simulink subsystem "aero_body_normal"  (R2026a)
settings: Solver=VariableStepAuto
undefined symbols (not defined in the file or in its folder): body_area_aft, body_area_bow, body_area_planform, body_length, body_pos_x_cp, body_volume, nosecone_area_aft, nosecone_area_bow, nosecone_area_planform, nosecone_length, nosecone_pos_x_cp, nosecone_volume, tail_area_aft, tail_area_bow, tail_area_planform, tail_length, tail_pos_x_cp, tail_volume
settings Model: Creator=joedo  LastModifiedBy=trist

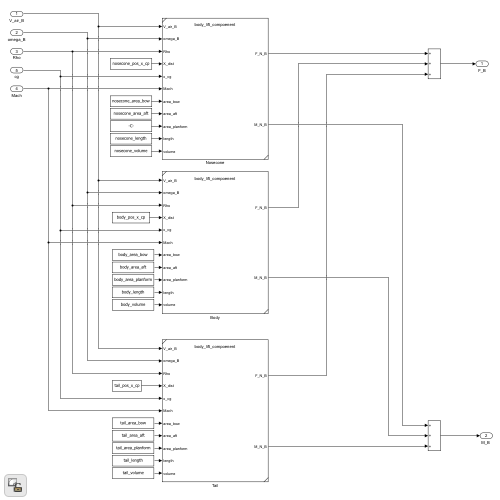
[thumbnail: Simulink's stored preview of the top-level diagram]
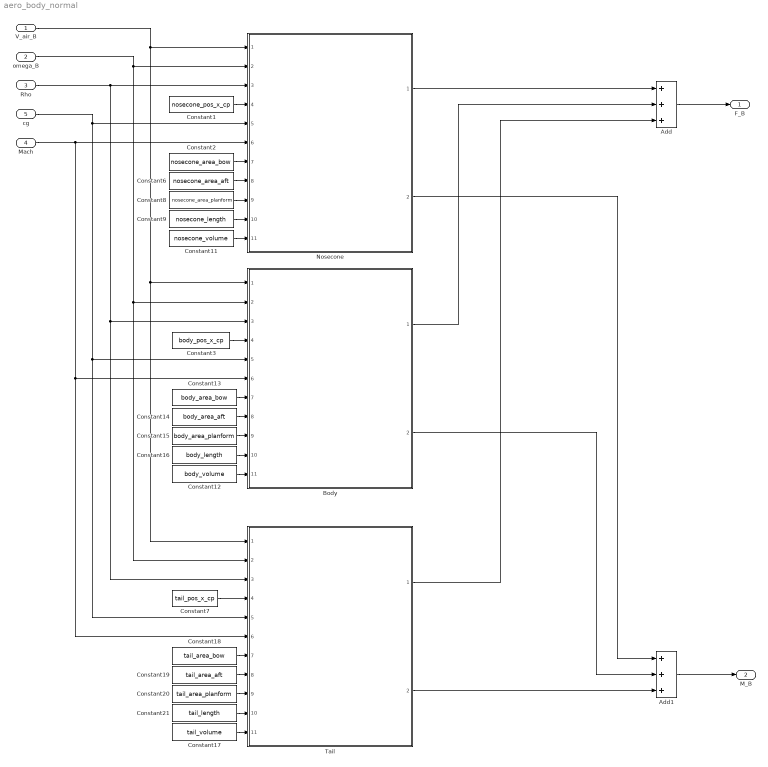
== system aero_body_normal ==
  "V_air_B " : Inport
  omega_B : Inport  Port=2
  Rho : Inport  Port=3
  Mach : Inport  Port=4
  cg : Inport  Port=5
  Add : Sum  Inputs=+++
  Add1 : Sum  Inputs=+++
  Body : Subsystem  ReferencedSubsystem=body_lift_compoenent
  Constant1 : Constant  Value=nosecone_pos_x_cp
  Constant11 : Constant  Value=nosecone_volume
  Constant12 : Constant  Value=body_volume
  Constant13 : Constant  Value=body_area_bow
  Constant14 : Constant  Value=body_area_aft
  Constant15 : Constant  Value=body_area_planform
  Constant16 : Constant  Value=body_length
  Constant17 : Constant  Value=tail_volume
  Constant18 : Constant  Value=tail_area_bow
  Constant19 : Constant  Value=tail_area_aft
  Constant2 : Constant  Value=nosecone_area_bow
  Constant20 : Constant  Value=tail_area_planform
  Constant21 : Constant  Value=tail_length
  Constant3 : Constant  Value=body_pos_x_cp
  Constant6 : Constant  Value=nosecone_area_aft
  Constant7 : Constant  Value=tail_pos_x_cp
  Constant8 : Constant  Value=nosecone_area_planform
  Constant9 : Constant  Value=nosecone_length
  Nosecone : Subsystem  ReferencedSubsystem=body_lift_compoenent
  Tail : Subsystem  ReferencedSubsystem=body_lift_compoenent
  "F_B " : Outport  VectorParamsAs1DForOutWhenUnconnected=off
  "M_B " : Outport  Port=2  VectorParamsAs1DForOutWhenUnconnected=off
  wires:
  Constant7/1 -> Tail/4
  Constant3/1 -> Body/4
  Nosecone/2 -> Add1/1
  Nosecone/1 -> Add/1
  Constant1/1 -> Nosecone/4
  Tail/2 -> Add1/3
  Tail/1 -> Add/3
  Body/2 -> Add1/2
  Body/1 -> Add/2
  Add/1 -> "F_B "/1
  Add1/1 -> "M_B "/1
  Rho/1 -> Nosecone/3, Body/3, Tail/3
  Mach/1 -> Nosecone/6, Body/6, Tail/6
  omega_B/1 -> Nosecone/2, Body/2, Tail/2
  "V_air_B "/1 -> Nosecone/1, Tail/1, Body/1
  cg/1 -> Nosecone/5, Body/5, Tail/5
  Constant2/1 -> Nosecone/7
  Constant6/1 -> Nosecone/8
  Constant8/1 -> Nosecone/9
  Constant9/1 -> Nosecone/10
  Constant11/1 -> Nosecone/11
  Constant15/1 -> Body/9
  Constant12/1 -> Body/11
  Constant13/1 -> Body/7
  Constant14/1 -> Body/8
  Constant16/1 -> Body/10
  Constant20/1 -> Tail/9
  Constant17/1 -> Tail/11
  Constant18/1 -> Tail/7
  Constant19/1 -> Tail/8
  Constant21/1 -> Tail/10
